simulink model "powertrain"  (R2024b)
settings: Solver=VariableStepAuto  StartTime=0.0  StopTime=10.0  RelTol=1e-3
model workspace (MAT data in the model file):
  eta_gearbox = 0.98
  eta_inverter = 1
(part 3 of 4)

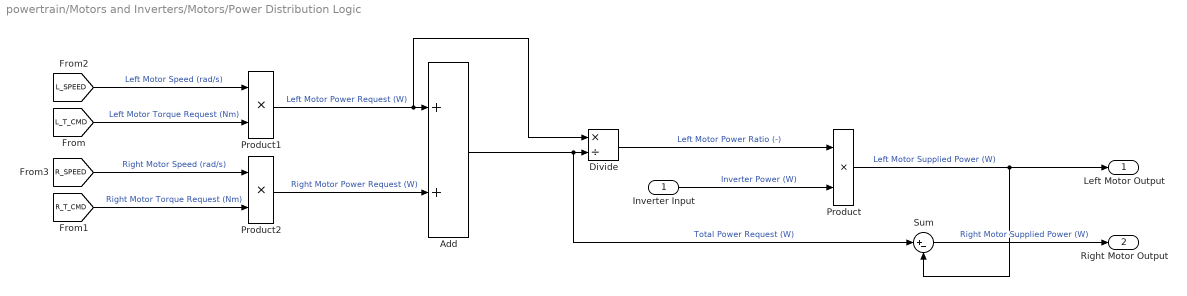
== system powertrain/Motors and Inverters/Motors/Power Distribution Logic ==
  Inverter Input : Inport
  Add : Sum
  Divide : Product  Inputs=*/
  Product : Product
  Product1 : Product
  Product2 : Product
  Sum : Sum  Inputs=|+-
  Left Motor Output : Outport
  Right Motor Output : Outport  Port=2
  wires:
  Inverter Input/1 -> Product/2  "Inverter Power (W)"
  Add/1 -> Sum/1, Divide/2  "Total Power Request (W)"
  Divide/1 -> Product/1  "Left Motor Power Ratio (-)"
  [L_SPEED] -> Product1/1  "Left Motor Speed (rad/s)"
  [L_T_CMD] -> Product1/2  "Left Motor Torque Request (Nm)"
  Product1/1 -> Divide/1, Add/1  "Left Motor Power Request (W)"
  [R_SPEED] -> Product2/1  "Right Motor Speed (rad/s)"
  [R_T_CMD] -> Product2/2  "Right Motor Torque Request (Nm)"
  Product2/1 -> Add/2  "Right Motor Power Request (W)"
  Product/1 -> Sum/2, Left Motor Output/1  "Left Motor Supplied Power (W)"
  Sum/1 -> Right Motor Output/1  "Right Motor Supplied Power (W)"
